simulink model "generate_proximity_sensor_re0"  (R2018a)
settings: Solver=VariableStepAuto  StartTime=0.0  StopTime=120  FixedStep=0.01  MaxStep=.001  RelTol=1e-3
settings Model: Creator=U500304  LastModifiedBy=Rafael
settings SolverCC: ZeroCrossAlgorithm=Adaptive
settings DataIOCC: SaveOutput=off  SaveTime=off
settings DebuggingCC: MaxConsecutiveZCsMsg=warning

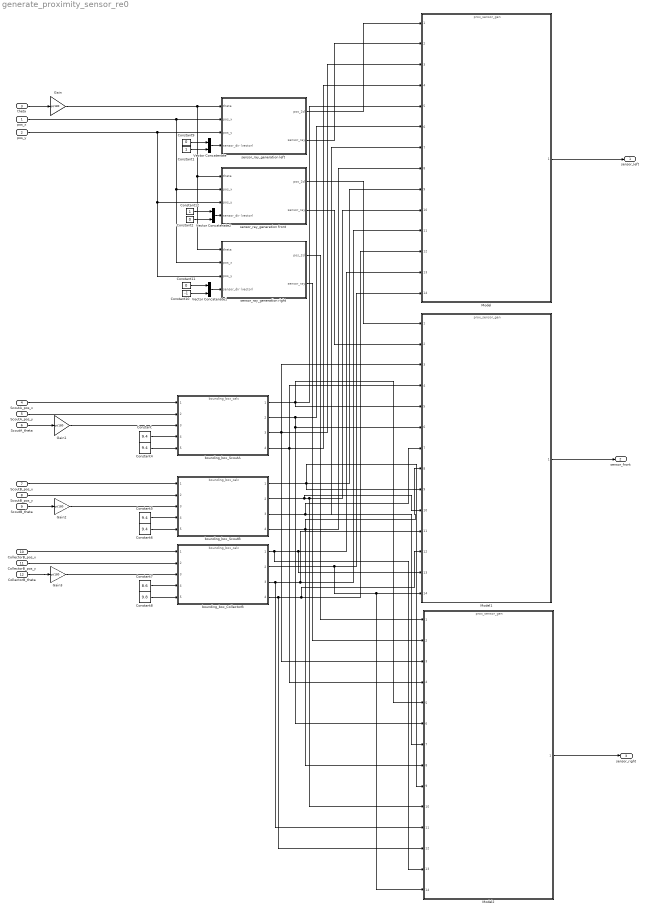
== system generate_proximity_sensor_re0 ==
  pos_x : Inport  OutDataTypeStr=double  PortDimensions=1  SampleTime=0
  pos_y : Inport  Port=2  OutDataTypeStr=double  PortDimensions=1  SampleTime=0
  theta : Inport  Port=3  OutDataTypeStr=double  PortDimensions=1  SampleTime=0
  ScoutA_pos_x : Inport  Port=4  OutDataTypeStr=double  PortDimensions=1  SampleTime=0
  ScoutA_pos_y : Inport  Port=5  OutDataTypeStr=double  PortDimensions=1  SampleTime=0
  ScoutA_theta : Inport  Port=6  OutDataTypeStr=double  PortDimensions=1  SampleTime=0
  ScoutB_pos_x : Inport  Port=7  OutDataTypeStr=double  PortDimensions=1  SampleTime=0
  ScoutB_pos_y : Inport  Port=8  OutDataTypeStr=double  PortDimensions=1  SampleTime=0
  ScoutB_theta : Inport  Port=9  OutDataTypeStr=double  PortDimensions=1  SampleTime=0
  CollectorB_pos_x : Inport  Port=10  OutDataTypeStr=double  PortDimensions=1  SampleTime=0
  CollectorB_pos_y : Inport  Port=11  OutDataTypeStr=double  PortDimensions=1  SampleTime=0
  CollectorB_theta : Inport  Port=12  OutDataTypeStr=double  PortDimensions=1  SampleTime=0
  Constant{,4..6} (4 alike) : Constant  Value=9.4
  Constant1 : Constant
  Constant10 : Constant  Value=-1
  Constant11 : Constant  Value=0
  Constant12 : Constant
  Constant2 : Constant  Value=0
  Constant7 : Constant  Value=8.6
  Constant8 : Constant  Value=9.8
  Constant9 : Constant  Value=0
  Gain{,1..3} (4 alike) : Gain  Gain=pi/180
  Model : ModelReference  ModelNameDialog=prox_sensor_gen  SimulationMode=Normal  ModelReferenceVersion=1.2
  Model1 : ModelReference  ModelNameDialog=prox_sensor_gen  SimulationMode=Normal  ModelReferenceVersion=1.2
  Model2 : ModelReference  ModelNameDialog=prox_sensor_gen  SimulationMode=Normal  ModelReferenceVersion=1.2
  Vector Concatenate : Concatenate
  Vector Concatenate1 : Concatenate
  Vector Concatenate2 : Concatenate
  bounding_box_CollectorB : ModelReference  ModelNameDialog=bounding_box_calc  SimulationMode=Normal  ModelReferenceVersion=1.659
  bounding_box_ScoutA : ModelReference  ModelNameDialog=bounding_box_calc  SimulationMode=Normal  ModelReferenceVersion=1.659
  bounding_box_ScoutB : ModelReference  ModelNameDialog=bounding_box_calc  SimulationMode=Normal  ModelReferenceVersion=1.659
  sensor_ray_generation front : Subsystem
  sensor_ray_generation left : Subsystem
  sensor_ray_generation right : Subsystem
  sensor_left : Outport  OutDataTypeStr=double  PortDimensions=1  SampleTime=0
  sensor_front : Outport  Port=2  OutDataTypeStr=double  PortDimensions=1  SampleTime=0
  "sensor_right " : Outport  Port=3  OutDataTypeStr=double  PortDimensions=1  SampleTime=0
  wires:
  theta/1 -> Gain/1
  bounding_box_CollectorB/2 -> Model1/14, Model2/14, Model/14
  Model2/1 -> "sensor_right "/1
  bounding_box_ScoutB/4 -> Model/8, Model1/8, Model2/8
  Constant8/1 -> bounding_box_CollectorB/5
  bounding_box_ScoutA/1 -> Model/5, Model1/5, Model2/5
  bounding_box_CollectorB/3 -> Model/11, Model1/11, Model2/11
  ScoutB_theta/1 -> Gain2/1
  Constant5/1 -> bounding_box_ScoutB/4
  ScoutA_pos_x/1 -> bounding_box_ScoutA/1
  bounding_box_ScoutA/3 -> Model1/3, Model2/3, Model/3
  Constant6/1 -> bounding_box_ScoutB/5
  Vector Concatenate/1 -> sensor_ray_generation left/4("sensor_dir (vector) ")
  bounding_box_CollectorB/1 -> Model/13, Model1/13, Model2/13
  bounding_box_ScoutA/4 -> Model1/4, Model2/4, Model/4
  sensor_ray_generation front/1(pos_2d) -> Model1/1
  sensor_ray_generation left/2("sensor_ray ") -> Model/2
  bounding_box_CollectorB/4 -> Model/12, Model1/12, Model2/12
  ScoutB_pos_y/1 -> bounding_box_ScoutB/2
  Model/1 -> sensor_left/1
  pos_y/1 -> sensor_ray_generation left/3(pos_y), sensor_ray_generation front/3(pos_y), sensor_ray_generation right/3(pos_y)
  bounding_box_ScoutB/2 -> Model/10, Model2/10, Model1/10
  Model1/1 -> sensor_front/1
  bounding_box_ScoutB/1 -> Model/9, Model1/9, Model2/9
  bounding_box_ScoutA/2 -> Model1/6, Model2/6, Model/6
  bounding_box_ScoutB/3 -> Model/7, Model1/7, Model2/7
  sensor_ray_generation right/2("sensor_ray ") -> Model2/2
  ScoutA_pos_y/1 -> bounding_box_ScoutA/2
  CollectorB_theta/1 -> Gain3/1
  pos_x/1 -> sensor_ray_generation left/2(pos_x), sensor_ray_generation front/2(pos_x), sensor_ray_generation right/2(pos_x)
  sensor_ray_generation right/1(pos_2d) -> Model2/1
  Constant4/1 -> bounding_box_ScoutA/5
  CollectorB_pos_x/1 -> bounding_box_CollectorB/1
  Constant/1 -> bounding_box_ScoutA/4
  CollectorB_pos_y/1 -> bounding_box_CollectorB/2
  Constant7/1 -> bounding_box_CollectorB/4
  ScoutA_theta/1 -> Gain1/1
  ScoutB_pos_x/1 -> bounding_box_ScoutB/1
  sensor_ray_generation left/1(pos_2d) -> Model/1
  sensor_ray_generation front/2("sensor_ray ") -> Model1/2
  Constant1/1 -> Vector Concatenate/2
  Constant9/1 -> Vector Concatenate/1
  Constant11/1 -> Vector Concatenate1/1
  Constant10/1 -> Vector Concatenate1/2
  Vector Concatenate1/1 -> sensor_ray_generation right/4("sensor_dir (vector) ")
  Vector Concatenate2/1 -> sensor_ray_generation front/4("sensor_dir (vector) ")
  Constant2/1 -> Vector Concatenate2/2
  Constant12/1 -> Vector Concatenate2/1
  Gain/1 -> sensor_ray_generation left/1("theta "), sensor_ray_generation front/1("theta "), sensor_ray_generation right/1("theta ")
  Gain1/1 -> bounding_box_ScoutA/3
  Gain2/1 -> bounding_box_ScoutB/3
  Gain3/1 -> bounding_box_CollectorB/3

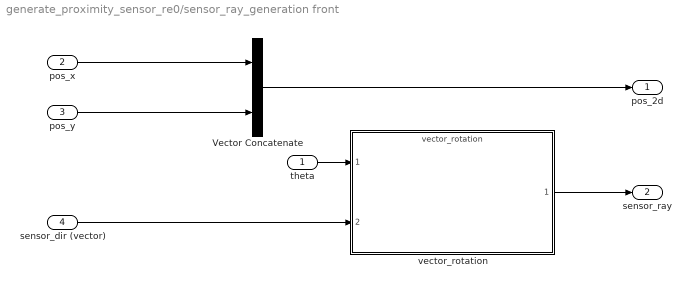
== system generate_proximity_sensor_re0/sensor_ray_generation front ==
  "theta " : Inport
  pos_x : Inport  Port=2
  pos_y : Inport  Port=3
  "sensor_dir (vector) " : Inport  Port=4
  Vector Concatenate : Concatenate
  vector_rotation : ModelReference  ModelNameDialog=vector_rotation  SimulationMode=Normal  ModelReferenceVersion=1.21
  pos_2d : Outport
  "sensor_ray " : Outport  Port=2
  wires:
  "sensor_dir (vector) "/1 -> vector_rotation/2
  "theta "/1 -> vector_rotation/1
  pos_x/1 -> Vector Concatenate/1
  Vector Concatenate/1 -> pos_2d/1
  pos_y/1 -> Vector Concatenate/2
  vector_rotation/1 -> "sensor_ray "/1

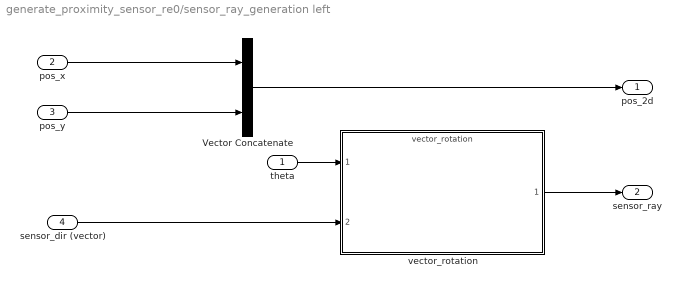
== system generate_proximity_sensor_re0/sensor_ray_generation left ==
  "theta " : Inport
  pos_x : Inport  Port=2
  pos_y : Inport  Port=3
  "sensor_dir (vector) " : Inport  Port=4
  Vector Concatenate : Concatenate
  vector_rotation : ModelReference  ModelNameDialog=vector_rotation  SimulationMode=Normal  ModelReferenceVersion=1.21
  pos_2d : Outport
  "sensor_ray " : Outport  Port=2
  wires:
  "sensor_dir (vector) "/1 -> vector_rotation/2
  vector_rotation/1 -> "sensor_ray "/1
  pos_y/1 -> Vector Concatenate/2
  Vector Concatenate/1 -> pos_2d/1
  pos_x/1 -> Vector Concatenate/1
  "theta "/1 -> vector_rotation/1

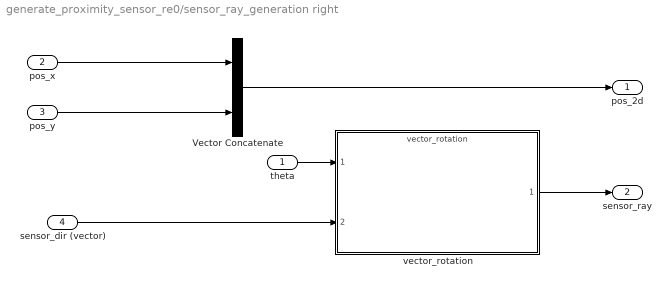
== system generate_proximity_sensor_re0/sensor_ray_generation right ==
  "theta " : Inport
  pos_x : Inport  Port=2
  pos_y : Inport  Port=3
  "sensor_dir (vector) " : Inport  Port=4
  Vector Concatenate : Concatenate
  vector_rotation : ModelReference  ModelNameDialog=vector_rotation  SimulationMode=Normal  ModelReferenceVersion=1.21
  pos_2d : Outport
  "sensor_ray " : Outport  Port=2
  wires:
  "theta "/1 -> vector_rotation/1
  "sensor_dir (vector) "/1 -> vector_rotation/2
  pos_x/1 -> Vector Concatenate/1
  Vector Concatenate/1 -> pos_2d/1
  pos_y/1 -> Vector Concatenate/2
  vector_rotation/1 -> "sensor_ray "/1
